simulink model "Hinf_control"  (R2017b)
settings: Solver=VariableStepAuto  StartTime=0.0  StopTime=3  RelTol=1e-3
undefined symbols (not defined in the file or in its folder): c_den, c_num, den, num
settings Model: Creator=hasee  LastModifiedBy=hasee

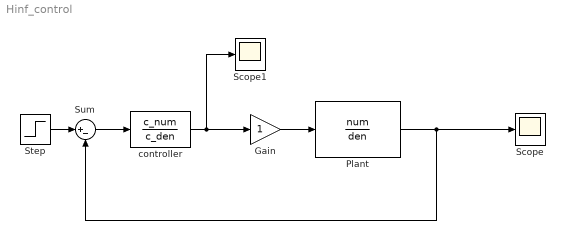
== system Hinf_control ==
  Gain : Gain
  Plant : TransferFcn  Numerator=num  Denominator=den
  Scope : Scope
  Scope1 : Scope
  Step : Step  SampleTime=0
  Sum : Sum  Inputs=|+-
  controller : TransferFcn  Numerator=c_num  Denominator=c_den
  wires:
  controller/1 -> Gain/1, Scope1/1
  Plant/1 -> Sum/2, Scope/1
  Step/1 -> Sum/1
  Sum/1 -> controller/1
  Gain/1 -> Plant/1
